simulink model "sl_subsys_fcncall8"  (Simulink 7.6)
settings: Solver=FixedStepDiscrete  StartTime=0.0  StopTime=10.0  FixedStep=1  RelTol=1e-3
undefined symbols (not defined in the file or in its folder): DiscIntNeverNeededParam
Description:
  | Function-call subsystems that specify periodic execution
  | 
  | The Stateflow chart below is used to schedule the execution order of function-call
  | subsystems in the model.  However, the function-call subsystems are executed
  | exactly once every time step.  The function calls are not used to specify
  | conditional execution, but rather simply to control the relative order of execution
  | of the subsystems.  This can be useful when data is transferred between the
  | subsystems using data stores, in order to ensure the proper sequence for reading
  | from and writing to the data stores.  Since the function-call subsystems are
  | intended to be executed unconditionally, we specify that they have a periodic
  | sample time (via the Sample time setting of the subsystems' TriggerPort blocks).
  | As a consequence, during simulation, the engine will verify that the
  | periodic function-call subsystems are indeed executed exactly once per time step.
  | In addition, when code is generated, elapsed time inside the function-call subsystems
  | is represented by a literal value (the specified, constant sample time) instead of
  | being maintained and computed from timers, as is standard for a function-call
  | subsystem.  Therefore the generated code is significantly more efficient.
  | 
  | Note the sample time color of the function-call subsystems is red rather than cyan,
  | indicating a periodic rather than triggered sample time. If the function-call
  | connections are interchanged, the result will be delayed one time step, due
  | to the modified interaction between the subsystems' data store read and write blocks.
settings Model: Creator=The MathWorks Inc.  CovMetricSettings=d  ExtModeAutoUpdateStatusClock=off
settings DataIOCC: SignalLoggingName=logsOut
settings OptimizationCC: BlockReduction=off  BooleanDataType=off  InlineInvariantSignals=on  InitFltsAndDblsToZero=on  OptimizeModelRefInitCode=on  LifeSpan=1
settings DebuggingCC: SaveWithParameterizedLinksMsg=none  CheckExecutionContextPreStartOutputMsg=on  CheckExecutionContextRuntimeOutputMsg=on  SignalResolutionControl=TryResolveAllWithWarning  SolverPrmCheckMsg=none  MultiTaskDSMMsg=warning  MultiTaskCondExecSysMsg=none
settings ModelReferenceCC: UpdateModelReferenceTargets=IfOutOfDate
settings SFSimCC: SimParseCustomCode=off
settings RTWCC: SystemTargetFile=ert.tlc  TemplateMakefile=ert_default_tmf  Description=RTW Embedded Coder (no auto configuration)  GenerateReport=on  ProcessScript=ert_make_rtw_hook  IncludeHyperlinkInReport=on  LaunchReport=on  IncludeERTFirstTime=on
settings CodeAppCC: IgnoreCustomStorageClasses=off  CustomSymbolStrFcn=$F$N$M
settings ERTTargetCC: TargetFcnLib=ansi_tfl_tmw.mat  MultiwordLength=2048  GenerateSampleERTMain=on  ERTCustomFileTemplate=example_file_process.tlc  ConvertIfToSwitch=off

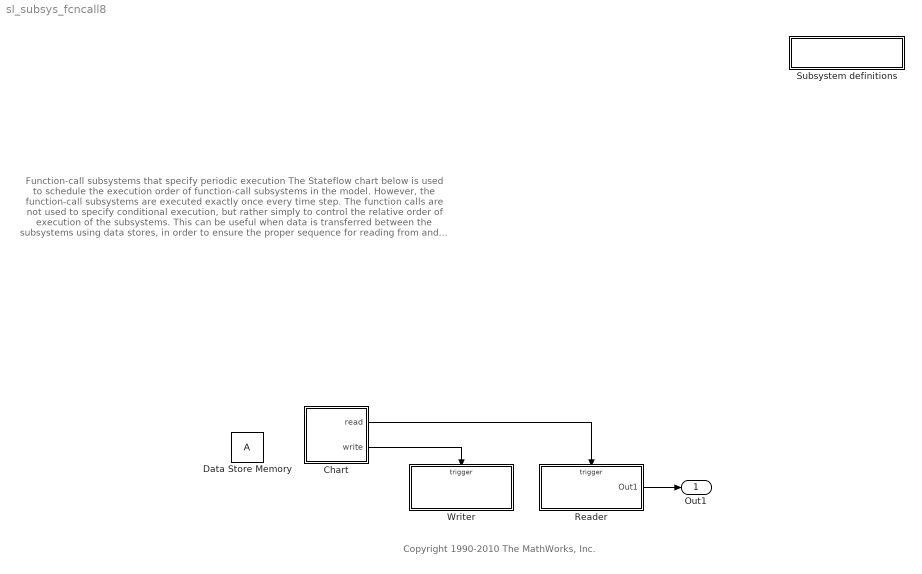
== system sl_subsys_fcncall8 ==
  note: Function-call subsystems that specify periodic execution
      |
      | The Stateflow chart below is used to schedule the execution order of function-call
      | subsystems in the model.  However, the function-call subsystems are executed
      | exactly once every time step.  The function calls are not used to specify
      | conditional execution, but rather simply to control the relative order of execution
      | of the subsystems.  This can be useful when data is transferred between the
      | subsystems using data stores, in order to ensure the proper sequence for reading
      | from and writing to the data stores.  Since the function-call subsystems are
      | intended to be executed unconditionally, we specify that they have a periodic
      | sample time (via the Sample time setting of the subsystems' TriggerPort blocks).
      | As a consequence, during simulation, the engine will verify that the
      | periodic function-call subsystems are indeed executed exactly once per time step.
      | In addition, when code is generated, elapsed time inside the function-call subsystems
      | is represented by a literal value (the specified, constant sample time) instead of
      | being maintained and computed from timers, as is standard for a function-call
      | subsystem.  Therefore the generated code is significantly more efficient.
      |
      | Note the sample time color of the function-call subsystems is red rather than cyan,
      | indicating a periodic rather than triggered sample time. If the function-call
      | connections are interchanged, the result will be delayed one time step, due
      | to the modified interaction between the subsystems' data store read and write blocks.
  note: Copyright 1990-2010 The MathWorks, Inc.
  " Subsystem definitions" : Subsystem
      settings: OpenFcn=helpview([matlabroot,'/toolbox/simulink/simdemos/simfeatures/html/sl_subsys_definitions.html']);
      mask Display: disp('Subsystem\ndefinitions')
  Chart : Stateflow chart  TreatAsAtomicUnit=on
  Data Store Memory : DataStoreMemory
  Reader : Subsystem  TreatAsAtomicUnit=on
  Writer : Subsystem  TreatAsAtomicUnit=on
  Out1 : Outport
  wires:
  Reader/1(Out1) -> Out1/1
  Chart/1(read) -> Reader/Trigger
  Chart/2(write) -> Writer/Trigger

== system sl_subsys_fcncall8/ Subsystem definitions ==

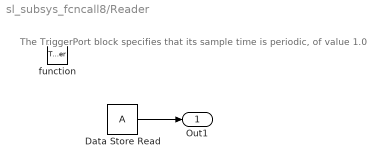
== system sl_subsys_fcncall8/Reader ==
  note: The TriggerPort block specifies that its
      | sample time is periodic, of value 1.0
  function : TriggerPort  TriggerType=function-call  SampleTimeType=periodic
  Data Store Read : DataStoreRead
  Out1 : Outport
  wires:
  Data Store Read/1 -> Out1/1

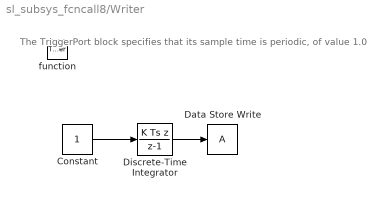
== system sl_subsys_fcncall8/Writer ==
  note: The TriggerPort block specifies that its
      | sample time is periodic, of value 1.0
  function : TriggerPort  TriggerType=function-call  SampleTimeType=periodic
  Constant : Constant
  Data Store Write : DataStoreWrite
  Discrete-Time Integrator : DiscreteIntegrator  IntegratorMethod=Integration: Backward Euler  SampleTime=-1  ICPrevOutput=DiscIntNeverNeededParam  ICPrevScaledInput=DiscIntNeverNeededParam
  wires:
  Constant/1 -> Discrete-Time Integrator/1
  Discrete-Time Integrator/1 -> Data Store Write/1

== stateflow chart Chart ==
  (default) -> (junction 3) : {write; read;}
  events: read output FUNCTION_CALL_EVENT; write output FUNCTION_CALL_EVENT
